simulink model "Charge_1_V1"  (R2017b)
settings: Solver=FixedStepDiscrete  StartTime=0.0  StopTime=1  FixedStep=0.001  RelTol=1e-3
PreLoadFcn:
  | librarySetup
  | eval([bdroot,'_startup']) %Calling [modelName]_startup.m
undefined symbols (not defined in the file or in its folder): A0, A1, Car1__Authorize, Car2_Authorize, CON2, CON3, CON4, Control_Mode_In, CurrentSP, D10, D12, D13, D2, D3, D4, D5, D6, D7, D8, Frequency_High_Point, Frequency_Low_Point, Frequency_Mid_high, Frequency_Mid_low, HVol_High_Point, HVol_Low_Point, HVol_Mid_high, HVol_Mid_low, HVoltage_Factor, SeconCar_ThreePhase, V_Current_five, V_Current_four, V_Current_one, V_Current_six, V_Current_three, V_Current_two, V_Frequency, V_MaxPliot, V_MinPliot, Vol_High_Point, Vol_Low_Point, Vol_Mid_high, Vol_Mid_low, Voltage_Factor, Voltage_Mode_Test
libraries: simulink x324, HANcoder_STM32_Target x30, powerlib_meascontrol x8, simulink_extras x2
(part 11 of 12)

== system Charge_1_V1/HANcoder STM32 Target - E407-STM32 algorithm/Energy Meter/Energy_Meter_Recieve/Subsystem1/Power_Meter/Current_phase2/Read_Gyro7 ==
  note: 01040000000271CB
  In1 : Inport
  Trigger : TriggerPort  VariantControl=Variant
  UART send : Subsystem  Tag=HANcoder_TARGET_STM32_E407  AncestorBlock=HANcoder_STM32_Target/STM32-E407/UART/UART send  mask(UART send){channel=UART1: CON3 - D1 & D0, useStatusOut=off, tsamp=-1}
      mask prompts: useStatusOut "Use status outport"; tsamp "Sample time"
      mask help:
      | Function
      | ==========
      | Transmits a byte on the UART communication interface.
      |
      | Parameters per channel
      | ======================
      | - Select channel (TX & RX)
      | - Select if the status output should be enabled.
      |
      | Inputs
      | ======
      | - The byte to send
      |
      | Outputs
      | =======
      | - When the status output is 0, the byte could not be transmitted. Probably
      |   because the transmit buffer was configured too small.
      mask init:
      | uartChannelInfoStr = sfcn_uart_send_mcb(2, channel, useStatusOut);
      settings: MoveFcn=drawLogos
      mask Help: web('sfcn_uart_send.html')
      mask TypeOptions channel: UART1: CON3 - D1 & D0 | UART2: CON PD - 8 & 9 | UART3: CON PD - 11 & 12 | UART6: UEXT - 3 & 4
      mask Display: fprintf('UART send\n%s', uartChannelInfoStr);patch([245 251 251],[8 14 2],[1 0 0]);patch([253 253 259],[14 2 8],[0 0 0.35]);
  wires:
  In1/1 -> UART send/1(In1)

== system Charge_1_V1/HANcoder STM32 Target - E407-STM32 algorithm/Energy Meter/Energy_Meter_Recieve/Subsystem1/Power_Meter/Current_phase2/Read_Gyro8 ==
  note: 01040000000271CB
  In1 : Inport
  Trigger : TriggerPort  VariantControl=Variant
  UART send : Subsystem  Tag=HANcoder_TARGET_STM32_E407  AncestorBlock=HANcoder_STM32_Target/STM32-E407/UART/UART send  mask(UART send){channel=UART1: CON3 - D1 & D0, useStatusOut=off, tsamp=-1}
      mask prompts: useStatusOut "Use status outport"; tsamp "Sample time"
      mask help:
      | Function
      | ==========
      | Transmits a byte on the UART communication interface.
      |
      | Parameters per channel
      | ======================
      | - Select channel (TX & RX)
      | - Select if the status output should be enabled.
      |
      | Inputs
      | ======
      | - The byte to send
      |
      | Outputs
      | =======
      | - When the status output is 0, the byte could not be transmitted. Probably
      |   because the transmit buffer was configured too small.
      mask init:
      | uartChannelInfoStr = sfcn_uart_send_mcb(2, channel, useStatusOut);
      settings: MoveFcn=drawLogos
      mask Help: web('sfcn_uart_send.html')
      mask TypeOptions channel: UART1: CON3 - D1 & D0 | UART2: CON PD - 8 & 9 | UART3: CON PD - 11 & 12 | UART6: UEXT - 3 & 4
      mask Display: fprintf('UART send\n%s', uartChannelInfoStr);patch([245 251 251],[8 14 2],[1 0 0]);patch([253 253 259],[14 2 8],[0 0 0.35]);
  wires:
  In1/1 -> UART send/1(In1)

== system Charge_1_V1/HANcoder STM32 Target - E407-STM32 algorithm/Energy Meter/Energy_Meter_Recieve/Subsystem1/Power_Meter/Current_phase2/Read_Gyro9 ==
  note: 01040000000271CB
  In1 : Inport
  Trigger : TriggerPort  VariantControl=Variant
  UART send : Subsystem  Tag=HANcoder_TARGET_STM32_E407  AncestorBlock=HANcoder_STM32_Target/STM32-E407/UART/UART send  mask(UART send){channel=UART1: CON3 - D1 & D0, useStatusOut=off, tsamp=-1}
      mask prompts: useStatusOut "Use status outport"; tsamp "Sample time"
      mask help:
      | Function
      | ==========
      | Transmits a byte on the UART communication interface.
      |
      | Parameters per channel
      | ======================
      | - Select channel (TX & RX)
      | - Select if the status output should be enabled.
      |
      | Inputs
      | ======
      | - The byte to send
      |
      | Outputs
      | =======
      | - When the status output is 0, the byte could not be transmitted. Probably
      |   because the transmit buffer was configured too small.
      mask init:
      | uartChannelInfoStr = sfcn_uart_send_mcb(2, channel, useStatusOut);
      settings: MoveFcn=drawLogos
      mask Help: web('sfcn_uart_send.html')
      mask TypeOptions channel: UART1: CON3 - D1 & D0 | UART2: CON PD - 8 & 9 | UART3: CON PD - 11 & 12 | UART6: UEXT - 3 & 4
      mask Display: fprintf('UART send\n%s', uartChannelInfoStr);patch([245 251 251],[8 14 2],[1 0 0]);patch([253 253 259],[14 2 8],[0 0 0.35]);
  wires:
  In1/1 -> UART send/1(In1)

== system Charge_1_V1/HANcoder STM32 Target - E407-STM32 algorithm/Energy Meter/Energy_Meter_Recieve/Subsystem1/Power_Meter/Last byte/UART send ==
  In1 : Inport
  Level-2 M-file S-Function : M-S-Function  FunctionName=sfcn_uart_send  Parameters=tsamp
  Term1 : Terminator
  wires:
  In1/1 -> Level-2 M-file S-Function/1
  Level-2 M-file S-Function/1 -> Term1/1

== system Charge_1_V1/HANcoder STM32 Target - E407-STM32 algorithm/Energy Meter/Energy_Meter_Recieve/Subsystem1/Power_Meter/Read_Gyro11/UART send ==
  In1 : Inport
  Level-2 M-file S-Function : M-S-Function  FunctionName=sfcn_uart_send  Parameters=tsamp
  Term1 : Terminator
  wires:
  In1/1 -> Level-2 M-file S-Function/1
  Level-2 M-file S-Function/1 -> Term1/1

== system Charge_1_V1/HANcoder STM32 Target - E407-STM32 algorithm/Energy Meter/Energy_Meter_Recieve/Subsystem1/Power_Meter/Read_Gyro6/UART send ==
  In1 : Inport
  Level-2 M-file S-Function : M-S-Function  FunctionName=sfcn_uart_send  Parameters=tsamp
  Term1 : Terminator
  wires:
  In1/1 -> Level-2 M-file S-Function/1
  Level-2 M-file S-Function/1 -> Term1/1

== system Charge_1_V1/HANcoder STM32 Target - E407-STM32 algorithm/Energy Meter/Energy_Meter_Recieve/Subsystem1/Power_Meter/Subsystem/Read_Gyro10 ==
  note: 01040000000271CB
  In1 : Inport
  Trigger : TriggerPort  VariantControl=Variant
  UART send : Subsystem  Tag=HANcoder_TARGET_STM32_E407  AncestorBlock=HANcoder_STM32_Target/STM32-E407/UART/UART send  mask(UART send){channel=UART1: CON3 - D1 & D0, useStatusOut=off, tsamp=-1}
      mask prompts: useStatusOut "Use status outport"; tsamp "Sample time"
      mask help:
      | Function
      | ==========
      | Transmits a byte on the UART communication interface.
      |
      | Parameters per channel
      | ======================
      | - Select channel (TX & RX)
      | - Select if the status output should be enabled.
      |
      | Inputs
      | ======
      | - The byte to send
      |
      | Outputs
      | =======
      | - When the status output is 0, the byte could not be transmitted. Probably
      |   because the transmit buffer was configured too small.
      mask init:
      | uartChannelInfoStr = sfcn_uart_send_mcb(2, channel, useStatusOut);
      settings: MoveFcn=drawLogos
      mask Help: web('sfcn_uart_send.html')
      mask TypeOptions channel: UART1: CON3 - D1 & D0 | UART2: CON PD - 8 & 9 | UART3: CON PD - 11 & 12 | UART6: UEXT - 3 & 4
      mask Display: fprintf('UART send\n%s', uartChannelInfoStr);patch([245 251 251],[8 14 2],[1 0 0]);patch([253 253 259],[14 2 8],[0 0 0.35]);
  wires:
  In1/1 -> UART send/1(In1)

== system Charge_1_V1/HANcoder STM32 Target - E407-STM32 algorithm/Energy Meter/Energy_Meter_Recieve/Subsystem1/Power_Meter/Subsystem/Read_Gyro12 ==
  note: 01040000000271CB
  In1 : Inport
  Trigger : TriggerPort  VariantControl=Variant
  UART send : Subsystem  Tag=HANcoder_TARGET_STM32_E407  AncestorBlock=HANcoder_STM32_Target/STM32-E407/UART/UART send  mask(UART send){channel=UART1: CON3 - D1 & D0, useStatusOut=off, tsamp=-1}
      mask prompts: useStatusOut "Use status outport"; tsamp "Sample time"
      mask help:
      | Function
      | ==========
      | Transmits a byte on the UART communication interface.
      |
      | Parameters per channel
      | ======================
      | - Select channel (TX & RX)
      | - Select if the status output should be enabled.
      |
      | Inputs
      | ======
      | - The byte to send
      |
      | Outputs
      | =======
      | - When the status output is 0, the byte could not be transmitted. Probably
      |   because the transmit buffer was configured too small.
      mask init:
      | uartChannelInfoStr = sfcn_uart_send_mcb(2, channel, useStatusOut);
      settings: MoveFcn=drawLogos
      mask Help: web('sfcn_uart_send.html')
      mask TypeOptions channel: UART1: CON3 - D1 & D0 | UART2: CON PD - 8 & 9 | UART3: CON PD - 11 & 12 | UART6: UEXT - 3 & 4
      mask Display: fprintf('UART send\n%s', uartChannelInfoStr);patch([245 251 251],[8 14 2],[1 0 0]);patch([253 253 259],[14 2 8],[0 0 0.35]);
  wires:
  In1/1 -> UART send/1(In1)

== system Charge_1_V1/HANcoder STM32 Target - E407-STM32 algorithm/Energy Meter/Energy_Meter_Recieve/Subsystem1/Power_Meter/Subsystem/Read_Gyro13 ==
  note: 01040000000271CB
  In1 : Inport
  Trigger : TriggerPort  VariantControl=Variant
  UART send : Subsystem  Tag=HANcoder_TARGET_STM32_E407  AncestorBlock=HANcoder_STM32_Target/STM32-E407/UART/UART send  mask(UART send){channel=UART1: CON3 - D1 & D0, useStatusOut=off, tsamp=-1}
      mask prompts: useStatusOut "Use status outport"; tsamp "Sample time"
      mask help:
      | Function
      | ==========
      | Transmits a byte on the UART communication interface.
      |
      | Parameters per channel
      | ======================
      | - Select channel (TX & RX)
      | - Select if the status output should be enabled.
      |
      | Inputs
      | ======
      | - The byte to send
      |
      | Outputs
      | =======
      | - When the status output is 0, the byte could not be transmitted. Probably
      |   because the transmit buffer was configured too small.
      mask init:
      | uartChannelInfoStr = sfcn_uart_send_mcb(2, channel, useStatusOut);
      settings: MoveFcn=drawLogos
      mask Help: web('sfcn_uart_send.html')
      mask TypeOptions channel: UART1: CON3 - D1 & D0 | UART2: CON PD - 8 & 9 | UART3: CON PD - 11 & 12 | UART6: UEXT - 3 & 4
      mask Display: fprintf('UART send\n%s', uartChannelInfoStr);patch([245 251 251],[8 14 2],[1 0 0]);patch([253 253 259],[14 2 8],[0 0 0.35]);
  wires:
  In1/1 -> UART send/1(In1)

== system Charge_1_V1/HANcoder STM32 Target - E407-STM32 algorithm/Energy Meter/Energy_Meter_Recieve/Subsystem1/Power_Meter/Subsystem/Read_Gyro14 ==
  note: 01040000000271CB
  In1 : Inport
  Trigger : TriggerPort  VariantControl=Variant
  UART send : Subsystem  Tag=HANcoder_TARGET_STM32_E407  AncestorBlock=HANcoder_STM32_Target/STM32-E407/UART/UART send  mask(UART send){channel=UART1: CON3 - D1 & D0, useStatusOut=off, tsamp=-1}
      mask prompts: useStatusOut "Use status outport"; tsamp "Sample time"
      mask help:
      | Function
      | ==========
      | Transmits a byte on the UART communication interface.
      |
      | Parameters per channel
      | ======================
      | - Select channel (TX & RX)
      | - Select if the status output should be enabled.
      |
      | Inputs
      | ======
      | - The byte to send
      |
      | Outputs
      | =======
      | - When the status output is 0, the byte could not be transmitted. Probably
      |   because the transmit buffer was configured too small.
      mask init:
      | uartChannelInfoStr = sfcn_uart_send_mcb(2, channel, useStatusOut);
      settings: MoveFcn=drawLogos
      mask Help: web('sfcn_uart_send.html')
      mask TypeOptions channel: UART1: CON3 - D1 & D0 | UART2: CON PD - 8 & 9 | UART3: CON PD - 11 & 12 | UART6: UEXT - 3 & 4
      mask Display: fprintf('UART send\n%s', uartChannelInfoStr);patch([245 251 251],[8 14 2],[1 0 0]);patch([253 253 259],[14 2 8],[0 0 0.35]);
  wires:
  In1/1 -> UART send/1(In1)

== system Charge_1_V1/HANcoder STM32 Target - E407-STM32 algorithm/Energy Meter/Energy_Meter_Recieve/Subsystem1/Power_Meter2/Current_Phase1/Read_Gyro1 ==
  note: 01040000000271CB
  In1 : Inport
  Trigger : TriggerPort  VariantControl=Variant
  UART send : Subsystem  Tag=HANcoder_TARGET_STM32_E407  AncestorBlock=HANcoder_STM32_Target/STM32-E407/UART/UART send  mask(UART send){channel=UART1: CON3 - D1 & D0, useStatusOut=off, tsamp=-1}
      mask prompts: useStatusOut "Use status outport"; tsamp "Sample time"
      mask help:
      | Function
      | ==========
      | Transmits a byte on the UART communication interface.
      |
      | Parameters per channel
      | ======================
      | - Select channel (TX & RX)
      | - Select if the status output should be enabled.
      |
      | Inputs
      | ======
      | - The byte to send
      |
      | Outputs
      | =======
      | - When the status output is 0, the byte could not be transmitted. Probably
      |   because the transmit buffer was configured too small.
      mask init:
      | uartChannelInfoStr = sfcn_uart_send_mcb(2, channel, useStatusOut);
      settings: MoveFcn=drawLogos
      mask Help: web('sfcn_uart_send.html')
      mask TypeOptions channel: UART1: CON3 - D1 & D0 | UART2: CON PD - 8 & 9 | UART3: CON PD - 11 & 12 | UART6: UEXT - 3 & 4
      mask Display: fprintf('UART send\n%s', uartChannelInfoStr);patch([245 251 251],[8 14 2],[1 0 0]);patch([253 253 259],[14 2 8],[0 0 0.35]);
  wires:
  In1/1 -> UART send/1(In1)

== system Charge_1_V1/HANcoder STM32 Target - E407-STM32 algorithm/Energy Meter/Energy_Meter_Recieve/Subsystem1/Power_Meter2/Current_Phase1/Read_Gyro2 ==
  note: 01040000000271CB
  In1 : Inport
  Trigger : TriggerPort  VariantControl=Variant
  UART send : Subsystem  Tag=HANcoder_TARGET_STM32_E407  AncestorBlock=HANcoder_STM32_Target/STM32-E407/UART/UART send  mask(UART send){channel=UART1: CON3 - D1 & D0, useStatusOut=off, tsamp=-1}
      mask prompts: useStatusOut "Use status outport"; tsamp "Sample time"
      mask help:
      | Function
      | ==========
      | Transmits a byte on the UART communication interface.
      |
      | Parameters per channel
      | ======================
      | - Select channel (TX & RX)
      | - Select if the status output should be enabled.
      |
      | Inputs
      | ======
      | - The byte to send
      |
      | Outputs
      | =======
      | - When the status output is 0, the byte could not be transmitted. Probably
      |   because the transmit buffer was configured too small.
      mask init:
      | uartChannelInfoStr = sfcn_uart_send_mcb(2, channel, useStatusOut);
      settings: MoveFcn=drawLogos
      mask Help: web('sfcn_uart_send.html')
      mask TypeOptions channel: UART1: CON3 - D1 & D0 | UART2: CON PD - 8 & 9 | UART3: CON PD - 11 & 12 | UART6: UEXT - 3 & 4
      mask Display: fprintf('UART send\n%s', uartChannelInfoStr);patch([245 251 251],[8 14 2],[1 0 0]);patch([253 253 259],[14 2 8],[0 0 0.35]);
  wires:
  In1/1 -> UART send/1(In1)

== system Charge_1_V1/HANcoder STM32 Target - E407-STM32 algorithm/Energy Meter/Energy_Meter_Recieve/Subsystem1/Power_Meter2/Current_Phase1/Read_Gyro3 ==
  note: 01040000000271CB
  In1 : Inport
  Trigger : TriggerPort  VariantControl=Variant
  UART send : Subsystem  Tag=HANcoder_TARGET_STM32_E407  AncestorBlock=HANcoder_STM32_Target/STM32-E407/UART/UART send  mask(UART send){channel=UART1: CON3 - D1 & D0, useStatusOut=off, tsamp=-1}
      mask prompts: useStatusOut "Use status outport"; tsamp "Sample time"
      mask help:
      | Function
      | ==========
      | Transmits a byte on the UART communication interface.
      |
      | Parameters per channel
      | ======================
      | - Select channel (TX & RX)
      | - Select if the status output should be enabled.
      |
      | Inputs
      | ======
      | - The byte to send
      |
      | Outputs
      | =======
      | - When the status output is 0, the byte could not be transmitted. Probably
      |   because the transmit buffer was configured too small.
      mask init:
      | uartChannelInfoStr = sfcn_uart_send_mcb(2, channel, useStatusOut);
      settings: MoveFcn=drawLogos
      mask Help: web('sfcn_uart_send.html')
      mask TypeOptions channel: UART1: CON3 - D1 & D0 | UART2: CON PD - 8 & 9 | UART3: CON PD - 11 & 12 | UART6: UEXT - 3 & 4
      mask Display: fprintf('UART send\n%s', uartChannelInfoStr);patch([245 251 251],[8 14 2],[1 0 0]);patch([253 253 259],[14 2 8],[0 0 0.35]);
  wires:
  In1/1 -> UART send/1(In1)

== system Charge_1_V1/HANcoder STM32 Target - E407-STM32 algorithm/Energy Meter/Energy_Meter_Recieve/Subsystem1/Power_Meter2/Current_Phase1/Read_Gyro4 ==
  note: 01040000000271CB
  In1 : Inport
  Trigger : TriggerPort  VariantControl=Variant
  UART send : Subsystem  Tag=HANcoder_TARGET_STM32_E407  AncestorBlock=HANcoder_STM32_Target/STM32-E407/UART/UART send  mask(UART send){channel=UART1: CON3 - D1 & D0, useStatusOut=off, tsamp=-1}
      mask prompts: useStatusOut "Use status outport"; tsamp "Sample time"
      mask help:
      | Function
      | ==========
      | Transmits a byte on the UART communication interface.
      |
      | Parameters per channel
      | ======================
      | - Select channel (TX & RX)
      | - Select if the status output should be enabled.
      |
      | Inputs
      | ======
      | - The byte to send
      |
      | Outputs
      | =======
      | - When the status output is 0, the byte could not be transmitted. Probably
      |   because the transmit buffer was configured too small.
      mask init:
      | uartChannelInfoStr = sfcn_uart_send_mcb(2, channel, useStatusOut);
      settings: MoveFcn=drawLogos
      mask Help: web('sfcn_uart_send.html')
      mask TypeOptions channel: UART1: CON3 - D1 & D0 | UART2: CON PD - 8 & 9 | UART3: CON PD - 11 & 12 | UART6: UEXT - 3 & 4
      mask Display: fprintf('UART send\n%s', uartChannelInfoStr);patch([245 251 251],[8 14 2],[1 0 0]);patch([253 253 259],[14 2 8],[0 0 0.35]);
  wires:
  In1/1 -> UART send/1(In1)

== system Charge_1_V1/HANcoder STM32 Target - E407-STM32 algorithm/Energy Meter/Energy_Meter_Recieve/Subsystem1/Power_Meter2/Current_phase2/Read_Gyro5 ==
  note: 01040000000271CB
  In1 : Inport
  Trigger : TriggerPort  VariantControl=Variant
  UART send : Subsystem  Tag=HANcoder_TARGET_STM32_E407  AncestorBlock=HANcoder_STM32_Target/STM32-E407/UART/UART send  mask(UART send){channel=UART1: CON3 - D1 & D0, useStatusOut=off, tsamp=-1}
      mask prompts: useStatusOut "Use status outport"; tsamp "Sample time"
      mask help:
      | Function
      | ==========
      | Transmits a byte on the UART communication interface.
      |
      | Parameters per channel
      | ======================
      | - Select channel (TX & RX)
      | - Select if the status output should be enabled.
      |
      | Inputs
      | ======
      | - The byte to send
      |
      | Outputs
      | =======
      | - When the status output is 0, the byte could not be transmitted. Probably
      |   because the transmit buffer was configured too small.
      mask init:
      | uartChannelInfoStr = sfcn_uart_send_mcb(2, channel, useStatusOut);
      settings: MoveFcn=drawLogos
      mask Help: web('sfcn_uart_send.html')
      mask TypeOptions channel: UART1: CON3 - D1 & D0 | UART2: CON PD - 8 & 9 | UART3: CON PD - 11 & 12 | UART6: UEXT - 3 & 4
      mask Display: fprintf('UART send\n%s', uartChannelInfoStr);patch([245 251 251],[8 14 2],[1 0 0]);patch([253 253 259],[14 2 8],[0 0 0.35]);
  wires:
  In1/1 -> UART send/1(In1)

== system Charge_1_V1/HANcoder STM32 Target - E407-STM32 algorithm/Energy Meter/Energy_Meter_Recieve/Subsystem1/Power_Meter2/Current_phase2/Read_Gyro7 ==
  note: 01040000000271CB
  In1 : Inport
  Trigger : TriggerPort  VariantControl=Variant
  UART send : Subsystem  Tag=HANcoder_TARGET_STM32_E407  AncestorBlock=HANcoder_STM32_Target/STM32-E407/UART/UART send  mask(UART send){channel=UART1: CON3 - D1 & D0, useStatusOut=off, tsamp=-1}
      mask prompts: useStatusOut "Use status outport"; tsamp "Sample time"
      mask help:
      | Function
      | ==========
      | Transmits a byte on the UART communication interface.
      |
      | Parameters per channel
      | ======================
      | - Select channel (TX & RX)
      | - Select if the status output should be enabled.
      |
      | Inputs
      | ======
      | - The byte to send
      |
      | Outputs
      | =======
      | - When the status output is 0, the byte could not be transmitted. Probably
      |   because the transmit buffer was configured too small.
      mask init:
      | uartChannelInfoStr = sfcn_uart_send_mcb(2, channel, useStatusOut);
      settings: MoveFcn=drawLogos
      mask Help: web('sfcn_uart_send.html')
      mask TypeOptions channel: UART1: CON3 - D1 & D0 | UART2: CON PD - 8 & 9 | UART3: CON PD - 11 & 12 | UART6: UEXT - 3 & 4
      mask Display: fprintf('UART send\n%s', uartChannelInfoStr);patch([245 251 251],[8 14 2],[1 0 0]);patch([253 253 259],[14 2 8],[0 0 0.35]);
  wires:
  In1/1 -> UART send/1(In1)

== system Charge_1_V1/HANcoder STM32 Target - E407-STM32 algorithm/Energy Meter/Energy_Meter_Recieve/Subsystem1/Power_Meter2/Current_phase2/Read_Gyro8 ==
  note: 01040000000271CB
  In1 : Inport
  Trigger : TriggerPort  VariantControl=Variant
  UART send : Subsystem  Tag=HANcoder_TARGET_STM32_E407  AncestorBlock=HANcoder_STM32_Target/STM32-E407/UART/UART send  mask(UART send){channel=UART1: CON3 - D1 & D0, useStatusOut=off, tsamp=-1}
      mask prompts: useStatusOut "Use status outport"; tsamp "Sample time"
      mask help:
      | Function
      | ==========
      | Transmits a byte on the UART communication interface.
      |
      | Parameters per channel
      | ======================
      | - Select channel (TX & RX)
      | - Select if the status output should be enabled.
      |
      | Inputs
      | ======
      | - The byte to send
      |
      | Outputs
      | =======
      | - When the status output is 0, the byte could not be transmitted. Probably
      |   because the transmit buffer was configured too small.
      mask init:
      | uartChannelInfoStr = sfcn_uart_send_mcb(2, channel, useStatusOut);
      settings: MoveFcn=drawLogos
      mask Help: web('sfcn_uart_send.html')
      mask TypeOptions channel: UART1: CON3 - D1 & D0 | UART2: CON PD - 8 & 9 | UART3: CON PD - 11 & 12 | UART6: UEXT - 3 & 4
      mask Display: fprintf('UART send\n%s', uartChannelInfoStr);patch([245 251 251],[8 14 2],[1 0 0]);patch([253 253 259],[14 2 8],[0 0 0.35]);
  wires:
  In1/1 -> UART send/1(In1)

== system Charge_1_V1/HANcoder STM32 Target - E407-STM32 algorithm/Energy Meter/Energy_Meter_Recieve/Subsystem1/Power_Meter2/Current_phase2/Read_Gyro9 ==
  note: 01040000000271CB
  In1 : Inport
  Trigger : TriggerPort  VariantControl=Variant
  UART send : Subsystem  Tag=HANcoder_TARGET_STM32_E407  AncestorBlock=HANcoder_STM32_Target/STM32-E407/UART/UART send  mask(UART send){channel=UART1: CON3 - D1 & D0, useStatusOut=off, tsamp=-1}
      mask prompts: useStatusOut "Use status outport"; tsamp "Sample time"
      mask help:
      | Function
      | ==========
      | Transmits a byte on the UART communication interface.
      |
      | Parameters per channel
      | ======================
      | - Select channel (TX & RX)
      | - Select if the status output should be enabled.
      |
      | Inputs
      | ======
      | - The byte to send
      |
      | Outputs
      | =======
      | - When the status output is 0, the byte could not be transmitted. Probably
      |   because the transmit buffer was configured too small.
      mask init:
      | uartChannelInfoStr = sfcn_uart_send_mcb(2, channel, useStatusOut);
      settings: MoveFcn=drawLogos
      mask Help: web('sfcn_uart_send.html')
      mask TypeOptions channel: UART1: CON3 - D1 & D0 | UART2: CON PD - 8 & 9 | UART3: CON PD - 11 & 12 | UART6: UEXT - 3 & 4
      mask Display: fprintf('UART send\n%s', uartChannelInfoStr);patch([245 251 251],[8 14 2],[1 0 0]);patch([253 253 259],[14 2 8],[0 0 0.35]);
  wires:
  In1/1 -> UART send/1(In1)

== system Charge_1_V1/HANcoder STM32 Target - E407-STM32 algorithm/Energy Meter/Energy_Meter_Recieve/Subsystem1/Power_Meter2/Last byte/UART send ==
  In1 : Inport
  Level-2 M-file S-Function : M-S-Function  FunctionName=sfcn_uart_send  Parameters=tsamp
  Term1 : Terminator
  wires:
  Level-2 M-file S-Function/1 -> Term1/1
  In1/1 -> Level-2 M-file S-Function/1

== system Charge_1_V1/HANcoder STM32 Target - E407-STM32 algorithm/Energy Meter/Energy_Meter_Recieve/Subsystem1/Power_Meter2/Read_Gyro11/UART send ==
  In1 : Inport
  Level-2 M-file S-Function : M-S-Function  FunctionName=sfcn_uart_send  Parameters=tsamp
  Term1 : Terminator
  wires:
  Level-2 M-file S-Function/1 -> Term1/1
  In1/1 -> Level-2 M-file S-Function/1

== system Charge_1_V1/HANcoder STM32 Target - E407-STM32 algorithm/Energy Meter/Energy_Meter_Recieve/Subsystem1/Power_Meter2/Read_Gyro6/UART send ==
  In1 : Inport
  Level-2 M-file S-Function : M-S-Function  FunctionName=sfcn_uart_send  Parameters=tsamp
  Term1 : Terminator
  wires:
  Level-2 M-file S-Function/1 -> Term1/1
  In1/1 -> Level-2 M-file S-Function/1

== system Charge_1_V1/HANcoder STM32 Target - E407-STM32 algorithm/Energy Meter/Energy_Meter_Recieve/Subsystem1/Power_Meter2/Subsystem/Read_Gyro10 ==
  note: 01040000000271CB
  In1 : Inport
  Trigger : TriggerPort  VariantControl=Variant
  UART send : Subsystem  Tag=HANcoder_TARGET_STM32_E407  AncestorBlock=HANcoder_STM32_Target/STM32-E407/UART/UART send  mask(UART send){channel=UART1: CON3 - D1 & D0, useStatusOut=off, tsamp=-1}
      mask prompts: useStatusOut "Use status outport"; tsamp "Sample time"
      mask help:
      | Function
      | ==========
      | Transmits a byte on the UART communication interface.
      |
      | Parameters per channel
      | ======================
      | - Select channel (TX & RX)
      | - Select if the status output should be enabled.
      |
      | Inputs
      | ======
      | - The byte to send
      |
      | Outputs
      | =======
      | - When the status output is 0, the byte could not be transmitted. Probably
      |   because the transmit buffer was configured too small.
      mask init:
      | uartChannelInfoStr = sfcn_uart_send_mcb(2, channel, useStatusOut);
      settings: MoveFcn=drawLogos
      mask Help: web('sfcn_uart_send.html')
      mask TypeOptions channel: UART1: CON3 - D1 & D0 | UART2: CON PD - 8 & 9 | UART3: CON PD - 11 & 12 | UART6: UEXT - 3 & 4
      mask Display: fprintf('UART send\n%s', uartChannelInfoStr);patch([245 251 251],[8 14 2],[1 0 0]);patch([253 253 259],[14 2 8],[0 0 0.35]);
  wires:
  In1/1 -> UART send/1(In1)

== system Charge_1_V1/HANcoder STM32 Target - E407-STM32 algorithm/Energy Meter/Energy_Meter_Recieve/Subsystem1/Power_Meter2/Subsystem/Read_Gyro12 ==
  note: 01040000000271CB
  In1 : Inport
  Trigger : TriggerPort  VariantControl=Variant
  UART send : Subsystem  Tag=HANcoder_TARGET_STM32_E407  AncestorBlock=HANcoder_STM32_Target/STM32-E407/UART/UART send  mask(UART send){channel=UART1: CON3 - D1 & D0, useStatusOut=off, tsamp=-1}
      mask prompts: useStatusOut "Use status outport"; tsamp "Sample time"
      mask help:
      | Function
      | ==========
      | Transmits a byte on the UART communication interface.
      |
      | Parameters per channel
      | ======================
      | - Select channel (TX & RX)
      | - Select if the status output should be enabled.
      |
      | Inputs
      | ======
      | - The byte to send
      |
      | Outputs
      | =======
      | - When the status output is 0, the byte could not be transmitted. Probably
      |   because the transmit buffer was configured too small.
      mask init:
      | uartChannelInfoStr = sfcn_uart_send_mcb(2, channel, useStatusOut);
      settings: MoveFcn=drawLogos
      mask Help: web('sfcn_uart_send.html')
      mask TypeOptions channel: UART1: CON3 - D1 & D0 | UART2: CON PD - 8 & 9 | UART3: CON PD - 11 & 12 | UART6: UEXT - 3 & 4
      mask Display: fprintf('UART send\n%s', uartChannelInfoStr);patch([245 251 251],[8 14 2],[1 0 0]);patch([253 253 259],[14 2 8],[0 0 0.35]);
  wires:
  In1/1 -> UART send/1(In1)

== system Charge_1_V1/HANcoder STM32 Target - E407-STM32 algorithm/Energy Meter/Energy_Meter_Recieve/Subsystem1/Power_Meter2/Subsystem/Read_Gyro13 ==
  note: 01040000000271CB
  In1 : Inport
  Trigger : TriggerPort  VariantControl=Variant
  UART send : Subsystem  Tag=HANcoder_TARGET_STM32_E407  AncestorBlock=HANcoder_STM32_Target/STM32-E407/UART/UART send  mask(UART send){channel=UART1: CON3 - D1 & D0, useStatusOut=off, tsamp=-1}
      mask prompts: useStatusOut "Use status outport"; tsamp "Sample time"
      mask help:
      | Function
      | ==========
      | Transmits a byte on the UART communication interface.
      |
      | Parameters per channel
      | ======================
      | - Select channel (TX & RX)
      | - Select if the status output should be enabled.
      |
      | Inputs
      | ======
      | - The byte to send
      |
      | Outputs
      | =======
      | - When the status output is 0, the byte could not be transmitted. Probably
      |   because the transmit buffer was configured too small.
      mask init:
      | uartChannelInfoStr = sfcn_uart_send_mcb(2, channel, useStatusOut);
      settings: MoveFcn=drawLogos
      mask Help: web('sfcn_uart_send.html')
      mask TypeOptions channel: UART1: CON3 - D1 & D0 | UART2: CON PD - 8 & 9 | UART3: CON PD - 11 & 12 | UART6: UEXT - 3 & 4
      mask Display: fprintf('UART send\n%s', uartChannelInfoStr);patch([245 251 251],[8 14 2],[1 0 0]);patch([253 253 259],[14 2 8],[0 0 0.35]);
  wires:
  In1/1 -> UART send/1(In1)

== system Charge_1_V1/HANcoder STM32 Target - E407-STM32 algorithm/Energy Meter/Energy_Meter_Recieve/Subsystem1/Power_Meter2/Subsystem/Read_Gyro14 ==
  note: 01040000000271CB
  In1 : Inport
  Trigger : TriggerPort  VariantControl=Variant
  UART send : Subsystem  Tag=HANcoder_TARGET_STM32_E407  AncestorBlock=HANcoder_STM32_Target/STM32-E407/UART/UART send  mask(UART send){channel=UART1: CON3 - D1 & D0, useStatusOut=off, tsamp=-1}
      mask prompts: useStatusOut "Use status outport"; tsamp "Sample time"
      mask help:
      | Function
      | ==========
      | Transmits a byte on the UART communication interface.
      |
      | Parameters per channel
      | ======================
      | - Select channel (TX & RX)
      | - Select if the status output should be enabled.
      |
      | Inputs
      | ======
      | - The byte to send
      |
      | Outputs
      | =======
      | - When the status output is 0, the byte could not be transmitted. Probably
      |   because the transmit buffer was configured too small.
      mask init:
      | uartChannelInfoStr = sfcn_uart_send_mcb(2, channel, useStatusOut);
      settings: MoveFcn=drawLogos
      mask Help: web('sfcn_uart_send.html')
      mask TypeOptions channel: UART1: CON3 - D1 & D0 | UART2: CON PD - 8 & 9 | UART3: CON PD - 11 & 12 | UART6: UEXT - 3 & 4
      mask Display: fprintf('UART send\n%s', uartChannelInfoStr);patch([245 251 251],[8 14 2],[1 0 0]);patch([253 253 259],[14 2 8],[0 0 0.35]);
  wires:
  In1/1 -> UART send/1(In1)

== system Charge_1_V1/HANcoder STM32 Target - E407-STM32 algorithm/Energy Meter/Energy_Meter_Recieve/Subsystem1/f/Current_Phase1/Read_Gyro1 ==
  note: 01040000000271CB
  In1 : Inport
  Trigger : TriggerPort  VariantControl=Variant
  UART send : Subsystem  Tag=HANcoder_TARGET_STM32_E407  AncestorBlock=HANcoder_STM32_Target/STM32-E407/UART/UART send  mask(UART send){channel=UART1: CON3 - D1 & D0, useStatusOut=off, tsamp=-1}
      mask prompts: useStatusOut "Use status outport"; tsamp "Sample time"
      mask help:
      | Function
      | ==========
      | Transmits a byte on the UART communication interface.
      |
      | Parameters per channel
      | ======================
      | - Select channel (TX & RX)
      | - Select if the status output should be enabled.
      |
      | Inputs
      | ======
      | - The byte to send
      |
      | Outputs
      | =======
      | - When the status output is 0, the byte could not be transmitted. Probably
      |   because the transmit buffer was configured too small.
      mask init:
      | uartChannelInfoStr = sfcn_uart_send_mcb(2, channel, useStatusOut);
      settings: MoveFcn=drawLogos
      mask Help: web('sfcn_uart_send.html')
      mask TypeOptions channel: UART1: CON3 - D1 & D0 | UART2: CON PD - 8 & 9 | UART3: CON PD - 11 & 12 | UART6: UEXT - 3 & 4
      mask Display: fprintf('UART send\n%s', uartChannelInfoStr);patch([245 251 251],[8 14 2],[1 0 0]);patch([253 253 259],[14 2 8],[0 0 0.35]);
  wires:
  In1/1 -> UART send/1(In1)

== system Charge_1_V1/HANcoder STM32 Target - E407-STM32 algorithm/Energy Meter/Energy_Meter_Recieve/Subsystem1/f/Current_Phase1/Read_Gyro2 ==
  note: 01040000000271CB
  In1 : Inport
  Trigger : TriggerPort  VariantControl=Variant
  UART send : Subsystem  Tag=HANcoder_TARGET_STM32_E407  AncestorBlock=HANcoder_STM32_Target/STM32-E407/UART/UART send  mask(UART send){channel=UART1: CON3 - D1 & D0, useStatusOut=off, tsamp=-1}
      mask prompts: useStatusOut "Use status outport"; tsamp "Sample time"
      mask help:
      | Function
      | ==========
      | Transmits a byte on the UART communication interface.
      |
      | Parameters per channel
      | ======================
      | - Select channel (TX & RX)
      | - Select if the status output should be enabled.
      |
      | Inputs
      | ======
      | - The byte to send
      |
      | Outputs
      | =======
      | - When the status output is 0, the byte could not be transmitted. Probably
      |   because the transmit buffer was configured too small.
      mask init:
      | uartChannelInfoStr = sfcn_uart_send_mcb(2, channel, useStatusOut);
      settings: MoveFcn=drawLogos
      mask Help: web('sfcn_uart_send.html')
      mask TypeOptions channel: UART1: CON3 - D1 & D0 | UART2: CON PD - 8 & 9 | UART3: CON PD - 11 & 12 | UART6: UEXT - 3 & 4
      mask Display: fprintf('UART send\n%s', uartChannelInfoStr);patch([245 251 251],[8 14 2],[1 0 0]);patch([253 253 259],[14 2 8],[0 0 0.35]);
  wires:
  In1/1 -> UART send/1(In1)

== system Charge_1_V1/HANcoder STM32 Target - E407-STM32 algorithm/Energy Meter/Energy_Meter_Recieve/Subsystem1/f/Current_Phase1/Read_Gyro3 ==
  note: 01040000000271CB
  In1 : Inport
  Trigger : TriggerPort  VariantControl=Variant
  UART send : Subsystem  Tag=HANcoder_TARGET_STM32_E407  AncestorBlock=HANcoder_STM32_Target/STM32-E407/UART/UART send  mask(UART send){channel=UART1: CON3 - D1 & D0, useStatusOut=off, tsamp=-1}
      mask prompts: useStatusOut "Use status outport"; tsamp "Sample time"
      mask help:
      | Function
      | ==========
      | Transmits a byte on the UART communication interface.
      |
      | Parameters per channel
      | ======================
      | - Select channel (TX & RX)
      | - Select if the status output should be enabled.
      |
      | Inputs
      | ======
      | - The byte to send
      |
      | Outputs
      | =======
      | - When the status output is 0, the byte could not be transmitted. Probably
      |   because the transmit buffer was configured too small.
      mask init:
      | uartChannelInfoStr = sfcn_uart_send_mcb(2, channel, useStatusOut);
      settings: MoveFcn=drawLogos
      mask Help: web('sfcn_uart_send.html')
      mask TypeOptions channel: UART1: CON3 - D1 & D0 | UART2: CON PD - 8 & 9 | UART3: CON PD - 11 & 12 | UART6: UEXT - 3 & 4
      mask Display: fprintf('UART send\n%s', uartChannelInfoStr);patch([245 251 251],[8 14 2],[1 0 0]);patch([253 253 259],[14 2 8],[0 0 0.35]);
  wires:
  In1/1 -> UART send/1(In1)

== system Charge_1_V1/HANcoder STM32 Target - E407-STM32 algorithm/Energy Meter/Energy_Meter_Recieve/Subsystem1/f/Current_Phase1/Read_Gyro4 ==
  note: 01040000000271CB
  In1 : Inport
  Trigger : TriggerPort  VariantControl=Variant
  UART send : Subsystem  Tag=HANcoder_TARGET_STM32_E407  AncestorBlock=HANcoder_STM32_Target/STM32-E407/UART/UART send  mask(UART send){channel=UART1: CON3 - D1 & D0, useStatusOut=off, tsamp=-1}
      mask prompts: useStatusOut "Use status outport"; tsamp "Sample time"
      mask help:
      | Function
      | ==========
      | Transmits a byte on the UART communication interface.
      |
      | Parameters per channel
      | ======================
      | - Select channel (TX & RX)
      | - Select if the status output should be enabled.
      |
      | Inputs
      | ======
      | - The byte to send
      |
      | Outputs
      | =======
      | - When the status output is 0, the byte could not be transmitted. Probably
      |   because the transmit buffer was configured too small.
      mask init:
      | uartChannelInfoStr = sfcn_uart_send_mcb(2, channel, useStatusOut);
      settings: MoveFcn=drawLogos
      mask Help: web('sfcn_uart_send.html')
      mask TypeOptions channel: UART1: CON3 - D1 & D0 | UART2: CON PD - 8 & 9 | UART3: CON PD - 11 & 12 | UART6: UEXT - 3 & 4
      mask Display: fprintf('UART send\n%s', uartChannelInfoStr);patch([245 251 251],[8 14 2],[1 0 0]);patch([253 253 259],[14 2 8],[0 0 0.35]);
  wires:
  In1/1 -> UART send/1(In1)

== system Charge_1_V1/HANcoder STM32 Target - E407-STM32 algorithm/Energy Meter/Energy_Meter_Recieve/Subsystem1/f/Current_phase2/Read_Gyro5 ==
  note: 01040000000271CB
  In1 : Inport
  Trigger : TriggerPort  VariantControl=Variant
  UART send : Subsystem  Tag=HANcoder_TARGET_STM32_E407  AncestorBlock=HANcoder_STM32_Target/STM32-E407/UART/UART send  mask(UART send){channel=UART1: CON3 - D1 & D0, useStatusOut=off, tsamp=-1}
      mask prompts: useStatusOut "Use status outport"; tsamp "Sample time"
      mask help:
      | Function
      | ==========
      | Transmits a byte on the UART communication interface.
      |
      | Parameters per channel
      | ======================
      | - Select channel (TX & RX)
      | - Select if the status output should be enabled.
      |
      | Inputs
      | ======
      | - The byte to send
      |
      | Outputs
      | =======
      | - When the status output is 0, the byte could not be transmitted. Probably
      |   because the transmit buffer was configured too small.
      mask init:
      | uartChannelInfoStr = sfcn_uart_send_mcb(2, channel, useStatusOut);
      settings: MoveFcn=drawLogos
      mask Help: web('sfcn_uart_send.html')
      mask TypeOptions channel: UART1: CON3 - D1 & D0 | UART2: CON PD - 8 & 9 | UART3: CON PD - 11 & 12 | UART6: UEXT - 3 & 4
      mask Display: fprintf('UART send\n%s', uartChannelInfoStr);patch([245 251 251],[8 14 2],[1 0 0]);patch([253 253 259],[14 2 8],[0 0 0.35]);
  wires:
  In1/1 -> UART send/1(In1)

== system Charge_1_V1/HANcoder STM32 Target - E407-STM32 algorithm/Energy Meter/Energy_Meter_Recieve/Subsystem1/f/Current_phase2/Read_Gyro7 ==
  note: 01040000000271CB
  In1 : Inport
  Trigger : TriggerPort  VariantControl=Variant
  UART send : Subsystem  Tag=HANcoder_TARGET_STM32_E407  AncestorBlock=HANcoder_STM32_Target/STM32-E407/UART/UART send  mask(UART send){channel=UART1: CON3 - D1 & D0, useStatusOut=off, tsamp=-1}
      mask prompts: useStatusOut "Use status outport"; tsamp "Sample time"
      mask help:
      | Function
      | ==========
      | Transmits a byte on the UART communication interface.
      |
      | Parameters per channel
      | ======================
      | - Select channel (TX & RX)
      | - Select if the status output should be enabled.
      |
      | Inputs
      | ======
      | - The byte to send
      |
      | Outputs
      | =======
      | - When the status output is 0, the byte could not be transmitted. Probably
      |   because the transmit buffer was configured too small.
      mask init:
      | uartChannelInfoStr = sfcn_uart_send_mcb(2, channel, useStatusOut);
      settings: MoveFcn=drawLogos
      mask Help: web('sfcn_uart_send.html')
      mask TypeOptions channel: UART1: CON3 - D1 & D0 | UART2: CON PD - 8 & 9 | UART3: CON PD - 11 & 12 | UART6: UEXT - 3 & 4
      mask Display: fprintf('UART send\n%s', uartChannelInfoStr);patch([245 251 251],[8 14 2],[1 0 0]);patch([253 253 259],[14 2 8],[0 0 0.35]);
  wires:
  In1/1 -> UART send/1(In1)

== system Charge_1_V1/HANcoder STM32 Target - E407-STM32 algorithm/Energy Meter/Energy_Meter_Recieve/Subsystem1/f/Current_phase2/Read_Gyro8 ==
  note: 01040000000271CB
  In1 : Inport
  Trigger : TriggerPort  VariantControl=Variant
  UART send : Subsystem  Tag=HANcoder_TARGET_STM32_E407  AncestorBlock=HANcoder_STM32_Target/STM32-E407/UART/UART send  mask(UART send){channel=UART1: CON3 - D1 & D0, useStatusOut=off, tsamp=-1}
      mask prompts: useStatusOut "Use status outport"; tsamp "Sample time"
      mask help:
      | Function
      | ==========
      | Transmits a byte on the UART communication interface.
      |
      | Parameters per channel
      | ======================
      | - Select channel (TX & RX)
      | - Select if the status output should be enabled.
      |
      | Inputs
      | ======
      | - The byte to send
      |
      | Outputs
      | =======
      | - When the status output is 0, the byte could not be transmitted. Probably
      |   because the transmit buffer was configured too small.
      mask init:
      | uartChannelInfoStr = sfcn_uart_send_mcb(2, channel, useStatusOut);
      settings: MoveFcn=drawLogos
      mask Help: web('sfcn_uart_send.html')
      mask TypeOptions channel: UART1: CON3 - D1 & D0 | UART2: CON PD - 8 & 9 | UART3: CON PD - 11 & 12 | UART6: UEXT - 3 & 4
      mask Display: fprintf('UART send\n%s', uartChannelInfoStr);patch([245 251 251],[8 14 2],[1 0 0]);patch([253 253 259],[14 2 8],[0 0 0.35]);
  wires:
  In1/1 -> UART send/1(In1)

== system Charge_1_V1/HANcoder STM32 Target - E407-STM32 algorithm/Energy Meter/Energy_Meter_Recieve/Subsystem1/f/Current_phase2/Read_Gyro9 ==
  note: 01040000000271CB
  In1 : Inport
  Trigger : TriggerPort  VariantControl=Variant
  UART send : Subsystem  Tag=HANcoder_TARGET_STM32_E407  AncestorBlock=HANcoder_STM32_Target/STM32-E407/UART/UART send  mask(UART send){channel=UART1: CON3 - D1 & D0, useStatusOut=off, tsamp=-1}
      mask prompts: useStatusOut "Use status outport"; tsamp "Sample time"
      mask help:
      | Function
      | ==========
      | Transmits a byte on the UART communication interface.
      |
      | Parameters per channel
      | ======================
      | - Select channel (TX & RX)
      | - Select if the status output should be enabled.
      |
      | Inputs
      | ======
      | - The byte to send
      |
      | Outputs
      | =======
      | - When the status output is 0, the byte could not be transmitted. Probably
      |   because the transmit buffer was configured too small.
      mask init:
      | uartChannelInfoStr = sfcn_uart_send_mcb(2, channel, useStatusOut);
      settings: MoveFcn=drawLogos
      mask Help: web('sfcn_uart_send.html')
      mask TypeOptions channel: UART1: CON3 - D1 & D0 | UART2: CON PD - 8 & 9 | UART3: CON PD - 11 & 12 | UART6: UEXT - 3 & 4
      mask Display: fprintf('UART send\n%s', uartChannelInfoStr);patch([245 251 251],[8 14 2],[1 0 0]);patch([253 253 259],[14 2 8],[0 0 0.35]);
  wires:
  In1/1 -> UART send/1(In1)

== system Charge_1_V1/HANcoder STM32 Target - E407-STM32 algorithm/Energy Meter/Energy_Meter_Recieve/Subsystem1/f/Current_phase3/Read_Gyro10 ==
  note: 01040000000271CB
  In1 : Inport
  Trigger : TriggerPort  VariantControl=Variant
  UART send : Subsystem  Tag=HANcoder_TARGET_STM32_E407  AncestorBlock=HANcoder_STM32_Target/STM32-E407/UART/UART send  mask(UART send){channel=UART1: CON3 - D1 & D0, useStatusOut=off, tsamp=-1}
      mask prompts: useStatusOut "Use status outport"; tsamp "Sample time"
      mask help:
      | Function
      | ==========
      | Transmits a byte on the UART communication interface.
      |
      | Parameters per channel
      | ======================
      | - Select channel (TX & RX)
      | - Select if the status output should be enabled.
      |
      | Inputs
      | ======
      | - The byte to send
      |
      | Outputs
      | =======
      | - When the status output is 0, the byte could not be transmitted. Probably
      |   because the transmit buffer was configured too small.
      mask init:
      | uartChannelInfoStr = sfcn_uart_send_mcb(2, channel, useStatusOut);
      settings: MoveFcn=drawLogos
      mask Help: web('sfcn_uart_send.html')
      mask TypeOptions channel: UART1: CON3 - D1 & D0 | UART2: CON PD - 8 & 9 | UART3: CON PD - 11 & 12 | UART6: UEXT - 3 & 4
      mask Display: fprintf('UART send\n%s', uartChannelInfoStr);patch([245 251 251],[8 14 2],[1 0 0]);patch([253 253 259],[14 2 8],[0 0 0.35]);
  wires:
  In1/1 -> UART send/1(In1)

== system Charge_1_V1/HANcoder STM32 Target - E407-STM32 algorithm/Energy Meter/Energy_Meter_Recieve/Subsystem1/f/Current_phase3/Read_Gyro12 ==
  note: 01040000000271CB
  In1 : Inport
  Trigger : TriggerPort  VariantControl=Variant
  UART send : Subsystem  Tag=HANcoder_TARGET_STM32_E407  AncestorBlock=HANcoder_STM32_Target/STM32-E407/UART/UART send  mask(UART send){channel=UART1: CON3 - D1 & D0, useStatusOut=off, tsamp=-1}
      mask prompts: useStatusOut "Use status outport"; tsamp "Sample time"
      mask help:
      | Function
      | ==========
      | Transmits a byte on the UART communication interface.
      |
      | Parameters per channel
      | ======================
      | - Select channel (TX & RX)
      | - Select if the status output should be enabled.
      |
      | Inputs
      | ======
      | - The byte to send
      |
      | Outputs
      | =======
      | - When the status output is 0, the byte could not be transmitted. Probably
      |   because the transmit buffer was configured too small.
      mask init:
      | uartChannelInfoStr = sfcn_uart_send_mcb(2, channel, useStatusOut);
      settings: MoveFcn=drawLogos
      mask Help: web('sfcn_uart_send.html')
      mask TypeOptions channel: UART1: CON3 - D1 & D0 | UART2: CON PD - 8 & 9 | UART3: CON PD - 11 & 12 | UART6: UEXT - 3 & 4
      mask Display: fprintf('UART send\n%s', uartChannelInfoStr);patch([245 251 251],[8 14 2],[1 0 0]);patch([253 253 259],[14 2 8],[0 0 0.35]);
  wires:
  In1/1 -> UART send/1(In1)

== system Charge_1_V1/HANcoder STM32 Target - E407-STM32 algorithm/Energy Meter/Energy_Meter_Recieve/Subsystem1/f/Current_phase3/Read_Gyro13 ==
  note: 01040000000271CB
  In1 : Inport
  Trigger : TriggerPort  VariantControl=Variant
  UART send : Subsystem  Tag=HANcoder_TARGET_STM32_E407  AncestorBlock=HANcoder_STM32_Target/STM32-E407/UART/UART send  mask(UART send){channel=UART1: CON3 - D1 & D0, useStatusOut=off, tsamp=-1}
      mask prompts: useStatusOut "Use status outport"; tsamp "Sample time"
      mask help:
      | Function
      | ==========
      | Transmits a byte on the UART communication interface.
      |
      | Parameters per channel
      | ======================
      | - Select channel (TX & RX)
      | - Select if the status output should be enabled.
      |
      | Inputs
      | ======
      | - The byte to send
      |
      | Outputs
      | =======
      | - When the status output is 0, the byte could not be transmitted. Probably
      |   because the transmit buffer was configured too small.
      mask init:
      | uartChannelInfoStr = sfcn_uart_send_mcb(2, channel, useStatusOut);
      settings: MoveFcn=drawLogos
      mask Help: web('sfcn_uart_send.html')
      mask TypeOptions channel: UART1: CON3 - D1 & D0 | UART2: CON PD - 8 & 9 | UART3: CON PD - 11 & 12 | UART6: UEXT - 3 & 4
      mask Display: fprintf('UART send\n%s', uartChannelInfoStr);patch([245 251 251],[8 14 2],[1 0 0]);patch([253 253 259],[14 2 8],[0 0 0.35]);
  wires:
  In1/1 -> UART send/1(In1)

== system Charge_1_V1/HANcoder STM32 Target - E407-STM32 algorithm/Energy Meter/Energy_Meter_Recieve/Subsystem1/f/Current_phase3/Read_Gyro14 ==
  note: 01040000000271CB
  In1 : Inport
  Trigger : TriggerPort  VariantControl=Variant
  UART send : Subsystem  Tag=HANcoder_TARGET_STM32_E407  AncestorBlock=HANcoder_STM32_Target/STM32-E407/UART/UART send  mask(UART send){channel=UART1: CON3 - D1 & D0, useStatusOut=off, tsamp=-1}
      mask prompts: useStatusOut "Use status outport"; tsamp "Sample time"
      mask help:
      | Function
      | ==========
      | Transmits a byte on the UART communication interface.
      |
      | Parameters per channel
      | ======================
      | - Select channel (TX & RX)
      | - Select if the status output should be enabled.
      |
      | Inputs
      | ======
      | - The byte to send
      |
      | Outputs
      | =======
      | - When the status output is 0, the byte could not be transmitted. Probably
      |   because the transmit buffer was configured too small.
      mask init:
      | uartChannelInfoStr = sfcn_uart_send_mcb(2, channel, useStatusOut);
      settings: MoveFcn=drawLogos
      mask Help: web('sfcn_uart_send.html')
      mask TypeOptions channel: UART1: CON3 - D1 & D0 | UART2: CON PD - 8 & 9 | UART3: CON PD - 11 & 12 | UART6: UEXT - 3 & 4
      mask Display: fprintf('UART send\n%s', uartChannelInfoStr);patch([245 251 251],[8 14 2],[1 0 0]);patch([253 253 259],[14 2 8],[0 0 0.35]);
  wires:
  In1/1 -> UART send/1(In1)

== system Charge_1_V1/HANcoder STM32 Target - E407-STM32 algorithm/Energy Meter/Energy_Meter_Recieve/Subsystem1/f/Last byte/UART send ==
  In1 : Inport
  Level-2 M-file S-Function : M-S-Function  FunctionName=sfcn_uart_send  Parameters=tsamp
  Term1 : Terminator
  wires:
  In1/1 -> Level-2 M-file S-Function/1
  Level-2 M-file S-Function/1 -> Term1/1

== system Charge_1_V1/HANcoder STM32 Target - E407-STM32 algorithm/Energy Meter/Energy_Meter_Recieve/Subsystem1/f/Read_Gyro11/UART send ==
  In1 : Inport
  Level-2 M-file S-Function : M-S-Function  FunctionName=sfcn_uart_send  Parameters=tsamp
  Term1 : Terminator
  wires:
  In1/1 -> Level-2 M-file S-Function/1
  Level-2 M-file S-Function/1 -> Term1/1

== system Charge_1_V1/HANcoder STM32 Target - E407-STM32 algorithm/Energy Meter/Energy_Meter_Recieve/Subsystem1/f/Read_Gyro6/UART send ==
  In1 : Inport
  Level-2 M-file S-Function : M-S-Function  FunctionName=sfcn_uart_send  Parameters=tsamp
  Term1 : Terminator
  wires:
  In1/1 -> Level-2 M-file S-Function/1
  Level-2 M-file S-Function/1 -> Term1/1

== system Charge_1_V1/HANcoder STM32 Target - E407-STM32 algorithm/Energy Meter/Energy_Meter_Recieve/Subsystem1/f1/Current_Phase1/Read_Gyro1 ==
  note: 01040000000271CB
  In1 : Inport
  Trigger : TriggerPort  VariantControl=Variant
  UART send : Subsystem  Tag=HANcoder_TARGET_STM32_E407  AncestorBlock=HANcoder_STM32_Target/STM32-E407/UART/UART send  mask(UART send){channel=UART1: CON3 - D1 & D0, useStatusOut=off, tsamp=-1}
      mask prompts: useStatusOut "Use status outport"; tsamp "Sample time"
      mask help:
      | Function
      | ==========
      | Transmits a byte on the UART communication interface.
      |
      | Parameters per channel
      | ======================
      | - Select channel (TX & RX)
      | - Select if the status output should be enabled.
      |
      | Inputs
      | ======
      | - The byte to send
      |
      | Outputs
      | =======
      | - When the status output is 0, the byte could not be transmitted. Probably
      |   because the transmit buffer was configured too small.
      mask init:
      | uartChannelInfoStr = sfcn_uart_send_mcb(2, channel, useStatusOut);
      settings: MoveFcn=drawLogos
      mask Help: web('sfcn_uart_send.html')
      mask TypeOptions channel: UART1: CON3 - D1 & D0 | UART2: CON PD - 8 & 9 | UART3: CON PD - 11 & 12 | UART6: UEXT - 3 & 4
      mask Display: fprintf('UART send\n%s', uartChannelInfoStr);patch([245 251 251],[8 14 2],[1 0 0]);patch([253 253 259],[14 2 8],[0 0 0.35]);
  wires:
  In1/1 -> UART send/1(In1)

== system Charge_1_V1/HANcoder STM32 Target - E407-STM32 algorithm/Energy Meter/Energy_Meter_Recieve/Subsystem1/f1/Current_Phase1/Read_Gyro2 ==
  note: 01040000000271CB
  In1 : Inport
  Trigger : TriggerPort  VariantControl=Variant
  UART send : Subsystem  Tag=HANcoder_TARGET_STM32_E407  AncestorBlock=HANcoder_STM32_Target/STM32-E407/UART/UART send  mask(UART send){channel=UART1: CON3 - D1 & D0, useStatusOut=off, tsamp=-1}
      mask prompts: useStatusOut "Use status outport"; tsamp "Sample time"
      mask help:
      | Function
      | ==========
      | Transmits a byte on the UART communication interface.
      |
      | Parameters per channel
      | ======================
      | - Select channel (TX & RX)
      | - Select if the status output should be enabled.
      |
      | Inputs
      | ======
      | - The byte to send
      |
      | Outputs
      | =======
      | - When the status output is 0, the byte could not be transmitted. Probably
      |   because the transmit buffer was configured too small.
      mask init:
      | uartChannelInfoStr = sfcn_uart_send_mcb(2, channel, useStatusOut);
      settings: MoveFcn=drawLogos
      mask Help: web('sfcn_uart_send.html')
      mask TypeOptions channel: UART1: CON3 - D1 & D0 | UART2: CON PD - 8 & 9 | UART3: CON PD - 11 & 12 | UART6: UEXT - 3 & 4
      mask Display: fprintf('UART send\n%s', uartChannelInfoStr);patch([245 251 251],[8 14 2],[1 0 0]);patch([253 253 259],[14 2 8],[0 0 0.35]);
  wires:
  In1/1 -> UART send/1(In1)
